simulink model "ClosedLoopControl"  (R2016b)
settings: Solver=FixedStepDiscrete  StartTime=0.0  StopTime=Inf  FixedStep=sCoreParams.core.stepPeriod  RelTol=1e-3  EnableMultiTasking=on
undefined symbols (not defined in the file): fdesignblkfcn, gcbh, High, sCoreParams, sCoreParams_decoders_chanceDetector_randStimEventsPerSec, sCoreParams_decoders_txDetector_channel1, sCoreParams_decoders_txDetector_channel2, sCoreParams_decoders_txDetector_detectChannelInds, sCoreParams_decoders_txDetector_nChannels, sCoreParams_Features_Baseline_initialThresholdValue, sCoreParams_Features_Baseline_weightPreviousThreshold, sCoreParams_Features_Data_SmoothWindowsDurationSamples, sCoreParams_stimulator_stimAfterDelaySteps
libraries: dsparch4 x20, dspstat3 x19, dspspect3 x6, dspfdesign x2, dspindex x2, dspswit3 x1
(part 4 of 6)

== system ClosedLoopControl/FilterBanks/Variant FILTER 1000/8-15Hz Alpha FIR ==
  EEGData : Inport
  Generated Filter Block : DiscreteFir  Tag=BlockMethodSubSystem  Coefficients=[1.1166843982614926e-06 -5.1505963497875887e-06 -1.2812602333555129e-05 -2.1871054990882468e-05 -3.2323373818540652e-05 -4.4162634838047868e-05 -5.7377540676991869e-05 -7.195240245586386e-05 -8.7867133639842035e-05 -0.00010509725598372113 -0.00012361391766630315 -0.00014338392367813367 -0.000164369778493665 -0.00018652974102566303 -0.00020981789182618625 -0.0002341842124648283 -0.0002595746769810637 -0.00028593135527383055 -0.00031319252825774447 -0.00034129281458180586 -0.00037016330867327857 -0.00039973172983648352 -0.00042992258210380332 -0.00046065732450443646 -0.00049185455138502153 -0.00052343018238589314 -0.000555297661646971 -0.0005873681657885076 -0.00061955082018408858 -0.00065175292301663287 -0.00068388017658249981 -0.00071583692528446631 -0.00074752639973140443 -0.00077885096634068161 -0.00080971238181931681 -0.00084001205188102607 -0.00086965129353934944 -0.00089853160030159028 -0.0009265549095744043 -0.00095362387157998788 -0.00097964211907159478 -0.0010045145371285577 -0.0010281475323047058 -0.0010504493003992363 -0.0010713300921165658 -0.0010907024758808866 -0.0011084815970723843 -0.0011245854329553625 -0.00113893504257369 -0.0011514548108961891 -0.001162072686503848 -0.0011707204121218695 -0.0011773337473127315 -0.0011818526826615754 -0.0011842216448022078 -0.0011843896916509528 -0.0011823106972363748 -0.0011779435255354414 -0.00117125219275111 -0.0011622060174923557 -0.0011507797583454361 -0.001136953738354511 -0.0011207139559606311 -0.0011020521819804436 -0.0010809660422397137 -0.001057459085511797 -0.0010315408364474827 -0.0010032268332200427 -0.00097253864964778316 -0.00093950390159584351 -0.00090415623749921738 -0.00086653531289007147 -0.00082668674885407638 -0.00078466207438273922 -0.00074051865263137029 -0.00069431959113537079 -0.0006461336360806941 -0.00059603505076769926 -0.00054410347845094465 -0.00049042378978056769 -0.0004350859151140158 -0.00037818466200922462 -0.0003198195182527428 -0.00026009444081761201 -0.00019911763118664756 -0.00013700129751690498 -7.3861404160011573e-05 -9.8174090911267554e-06 5.5008010163797022e-05 0.00012048924147724876 0.00018649803328639865 0.00025290379928409514 0.00031957393191114501 0.00038637412389685354 0.00045316869706702476 0.00051982093761261162 0.00058619343698820684 0.00065214843758748075 0.00071754818232275524 0.00078225526721801533 0.00084613299610908864 0.00090904573653135254 0.00097085927586427958 0.0010314411767934721 0.0010906611311446244 0.0011483913111399052 0.0012045067171260633 0.0012588855208245753 0.0013114094031579228 0.0013619638857121615 0.0014104386549047448 0.0014567278779377545 0.0015007305096304167 0.0015423505892410412 0.0015814975264072709 0.001618086375354588 0.0016520380965466808 0.0016832798049771526 0.0017117450043303123 0.0017373738062692796 0.0017601131341423238 0.0017799169104332252 0.0017967462273182613 0.0018105694997313348 0.0018213626003794627 0.0018291089761933916 0.0018337997457423454 0.0018354337771877447 0.0018340177463980255 0.0018295661748954481 0.0018221014473556757 0.0018116538084320456 0.0017982613387285684 0.0017819699097986867 0.0017628331181006056 0.0017409121978943678 0.0017162759131207782 0.0016890004283574528 0.0016591691590027344 0.0016268726008937253 0.001592208139620101 0.0015552798398505627 0.0015161982150436648 0.0014750799779690521 0.0014320477725188181 0.0013872298873415828 0.0013407599518838245 0.0012927766154738488 0.001243423210133381 0.0011928473978500983 0.0011412008030911467 0.0010886386313827949 0.0010353192748249133 0.00098140390545031655 0.0009270560573785804 0.00087244119875139019 0.00081772629447154682 0.00076307936080061199 0.00070866901290059193 0.00065466400643282975 0.00060123277435255879 0.00054854296006001896 0.00049676094808876381 0.00044605139352870261 0.00039657675139517979 0.00034849680716653192 0.0003019682097202846 0.00025714400790310016 0.00021417319197122785 0.00017320024113676101 0.00013436467845048239 9.7800634244212941e-05 6.3636419344704006e-05 3.1994109256920648e-05 ...(+13836 chars)]  InputProcessing=Columns as channels (frame based)
  filteredData : Outport
  wires:
  EEGData/1 -> Generated Filter Block/1
  Generated Filter Block/1 -> filteredData/1

== system ClosedLoopControl/FilterBanks/Variant FILTER 1000/8-15Hz Alpha IIR ==
  EEGData : Inport
  Generated Filter Block : dsparch4/Biquad Filter  Tag=BlockMethodSubSystem  IIRFiltStruct=Direct form II  CoeffSource=Specify via dialog  BiQuadCoeffs=[0.03152382825305871 0 -0.03152382825305871 1 -1.9684345944585124 0.97712907102407076;0.025560463242853482 0 -0.025560463242853482 1 -1.9681378422909206 0.97119496912467995;0.024051049006500725 0 -0.024051049006500725 1 -1.9527425358453594 0.95696285762488253;0.007268915115754877 0 -0.007268915115754877 1 -1.9493011946808791 0.95637402951036332;0.026129757567963516 0 -0.026129757567963516 1 -1.9934192573086764 0.99586503566620033;0.017980975322089195 0 -0.017980975322089195 1 -1.9829215784521332 0.99203325429180822;0.032745837103951347 0 -0.032745837103951347 1 -1.9568602017984618 0.9648466951679141;0.029923094077486778 0 -0.029923094077486778 1 -1.9599295286379477 0.96347484474396472;0.027004967888092691 0 -0.027004967888092691 1 -1.9477670142381809 0.95284532685210388;0.032600500740339038 0 -0.032600500740339038 1 -1.9463207424125604 0.9523841483440838;0.01817150925319717 0 -0.01817150925319717 1 -1.9850778884335281 0.98761149045414087;2 0 -2 1 -1.9766276718191218 0.97935766676512392]  a0Flag=Warning  IC=0  ICnum=0  ICden=0  InputProcessing=Columns as channels (frame based)  denAccumFracLength=30  denProdOutputFracLength=30  secondMemoryFracLength=15  roundingMode=Floor  overflowMode=off  ScaleValues=[0.0021262776362185819;1;1;1;1;1;1;1;1;1;1;1;4.7772804403775435]  optimizeScaleValues=off  ScaleValueMode=Specify via input port (g)  scaleValueFracLength=14  FilterSource=Specify via dialog  FilterObject=BQF
  filteredData : Outport
  wires:
  EEGData/1 -> Generated Filter Block/1
  Generated Filter Block/1 -> filteredData/1

== system ClosedLoopControl/FilterBanks/Variant FILTER 1000/80-200Hz HFORipple FIR ==
  EEGData : Inport
  Generated Filter Block : DiscreteFir  Tag=BlockMethodSubSystem  Coefficients=[-0.029929468383316192 0.027584903344857116 0.006558984880081789 -0.0071603267655065833 -0.013247180355273648 -0.013135920645701411 -0.0090343519140387157 -0.0032754151064268641 0.0022272516299482945 0.0061526392461596219 0.0079390912269469774 0.0076686887032404866 0.0060227556600073798 0.0039349955485136062 0.002396304305429954 0.0020527359637715833 0.0031029488412524647 0.0051247167458305515 0.0073477544104056103 0.0087957682525686351 0.0088043284423398316 0.00710059570242208 0.0041318613604908808 0.00067350576530127854 -0.0021332528816080248 -0.0036147405910317496 -0.0034016416976209995 -0.001904243925895048 -9.8116221945575288e-05 0.0011838227951950983 0.0010052402801807789 -0.00069375398602379568 -0.0033161108088197999 -0.0058093921651041838 -0.0070688296122434977 -0.0062279411320784531 -0.0032465358048272691 0.0011033746367409905 0.0054903794295953143 0.0085941785365106216 0.0095047981352248956 0.0081292793472463598 0.005237259579484288 0.0022388728520793405 0.00053886046527349546 0.00096339401712913775 0.0033698853216399469 0.006695473988653354 0.0093294470183197739 0.009730061973901652 0.0070986567584101143 0.0017181031971334401 -0.0049383095140956221 -0.010887765954854724 -0.014221289453944019 -0.013976819805220315 -0.010530893082807774 -0.0054287582554014349 -0.00088011910410184385 0.0011679539587099719 -0.00014547643883787431 -0.0041760754011632081 -0.008944366661674398 -0.011801424674010449 -0.010562162379392094 -0.0044555321547889229 0.0053958544645990661 0.016263138140394436 0.024694650965907963 0.027841496662202841 0.024596298085779726 0.016203929024829047 0.0058734470287940752 -0.0023244041555813555 -0.0050790680728182019 -0.0012630785826390906 0.0072633206754821183 0.016070445540513408 0.019596048919655211 0.013222985157710941 -0.0046438574372398012 -0.031492102130720984 -0.060763349522214613 -0.083541115124259574 -0.09120184118086383 -0.078307752643135484 -0.04470543854444764 0.0038254224665319886 0.056784017626830177 0.10164096275331343 0.12730747905853101 0.12730747905853101 0.10164096275331343 0.056784017626830177 0.0038254224665319886 -0.04470543854444764 -0.078307752643135484 -0.09120184118086383 -0.083541115124259574 -0.060763349522214613 -0.031492102130720984 -0.0046438574372398012 0.013222985157710941 0.019596048919655211 0.016070445540513408 0.0072633206754821183 -0.0012630785826390906 -0.0050790680728182019 -0.0023244041555813555 0.0058734470287940752 0.016203929024829047 0.024596298085779726 0.027841496662202841 0.024694650965907963 0.016263138140394436 0.0053958544645990661 -0.0044555321547889229 -0.010562162379392094 -0.011801424674010449 -0.008944366661674398 -0.0041760754011632081 -0.00014547643883787431 0.0011679539587099719 -0.00088011910410184385 -0.0054287582554014349 -0.010530893082807774 -0.013976819805220315 -0.014221289453944019 -0.010887765954854724 -0.0049383095140956221 0.0017181031971334401 0.0070986567584101143 0.009730061973901652 0.0093294470183197739 0.006695473988653354 0.0033698853216399469 0.00096339401712913775 0.00053886046527349546 0.0022388728520793405 0.005237259579484288 0.0081292793472463598 0.0095047981352248956 0.0085941785365106216 0.0054903794295953143 0.0011033746367409905 -0.0032465358048272691 -0.0062279411320784531 -0.0070688296122434977 -0.0058093921651041838 -0.0033161108088197999 -0.00069375398602379568 0.0010052402801807789 0.0011838227951950983 -9.8116221945575288e-05 -0.001904243925895048 -0.0034016416976209995 -0.0036147405910317496 -0.0021332528816080248 0.00067350576530127854 0.0041318613604908808 0.00710059570242208 0.0088043284423398316 0.0087957682525686351 0.0073477544104056103 0.0051247167458305515 0.0031029488412524647 0.0020527359637715833 0.002396304305429954 0.0039349955485136062 0.0060227556600073798 0.0076686887032404866 0.0079390912269469774 0.0061526392461596219 0.0022272516299482945 -0.0032754151064268641 -0.0090343519140387157 -0.013135920645701411 -0.013247180355273648 -0.0071603267655065833 0.006558984880081789 0.027584903344857116 -0.029929468383316192]  InputProcessing=Columns as channels (frame based)
  filteredData : Outport
  wires:
  EEGData/1 -> Generated Filter Block/1
  Generated Filter Block/1 -> filteredData/1

== system ClosedLoopControl/FilterBanks/Variant FILTER 1000/80-200Hz HFORipple IIR ==
  EEGData : Inport
  Generated Filter Block : dsparch4/Biquad Filter  Tag=BlockMethodSubSystem  IIRFiltStruct=Direct form II  CoeffSource=Specify via dialog  BiQuadCoeffs=[0.50528002861034449 0 -0.50528002861034449 1 -0.53665660289882711 0.75825785021660019;0.37399875098270552 0 -0.37399875098270552 1 -1.4711915314319288 0.71332426960135642;0.32821275057331467 0 -0.32821275057331467 1 -1.0345186757915159 0.43765324877783934;0.29499676491259791 0 -0.29499676491259791 1 -0.69551179724291168 0.41191642538380135;0.32493798324944001 0 -0.32493798324944001 1 -1.2744782347700396 0.5651630856467672;0.12068212430570054 0 -0.12068212430570054 1 -0.57105344445275907 0.53488062009913828;0.30353084173161105 0 -0.30353084173161105 1 -1.7216581336938179 0.9551476738605682;0.49261556542327029 0 -0.49261556542327029 1 -0.55816431380313891 0.91150109211215435;0.18405150815598884 0 -0.18405150815598884 1 -1.3775879521174472 0.63826277797818964;0.38868856803283353 0 -0.38868856803283353 1 -0.54207706836534775 0.63362507430418646;0.35661452914905484 0 -0.35661452914905484 1 -0.90735390108977221 0.39967170660663376;0.43873431466398466 0 -0.43873431466398466 1 -0.79136443478105378 0.39064255793275482;0.28072258344311274 0 -0.28072258344311274 1 -1.1597022390795022 0.49621962903073175;0.54469763526328785 0 -0.54469763526328785 1 -0.62218168437391907 0.46078823772386801;0.27221303222116677 0 -0.27221303222116677 1 -1.6408415799416185 0.87038248002913765;0.99524691708840851 0 -0.99524691708840851 1 -1.5580903198942666 0.79034416212980196]  a0Flag=Warning  IC=0  ICnum=0  ICden=0  InputProcessing=Columns as channels (frame based)  denAccumFracLength=30  denProdOutputFracLength=30  secondMemoryFracLength=15  roundingMode=Floor  overflowMode=off  ScaleValues=[0.22997867729739599;1;1;1;1;1;1;1;1;1;1;1;1;1;1;1;1]  optimizeScaleValues=off  ScaleValueMode=Specify via input port (g)  scaleValueFracLength=14  FilterSource=Specify via dialog  FilterObject=BQF
  filteredData : Outport
  wires:
  EEGData/1 -> Generated Filter Block/1
  Generated Filter Block/1 -> filteredData/1

== system ClosedLoopControl/FilterBanks/Variant FILTER 1000/AllBand ==
  EEGData : Inport
  filteredData : Outport
  wires:
  EEGData/1 -> filteredData/1

== system ClosedLoopControl/FilterBanks/Variant FILTER 1000/VariableFreq FIR ==
  EEGData : Inport
  Discrete FIR Filter : DiscreteFir  FilterStructure=Direct form symmetric  Coefficients=sCoreParams.filter.Hd.Numerator
  filteredData : Outport
  wires:
  Discrete FIR Filter/1 -> filteredData/1
  EEGData/1 -> Discrete FIR Filter/1

== system ClosedLoopControl/FilterBanks/Variant FILTER 2000/11-15HZ Spindles IIR ==
  EEGData : Inport
  Generated Filter Block : dsparch4/Biquad Filter  Tag=BlockMethodSubSystem  IIRFiltStruct=Direct form II  CoeffSource=Specify via dialog  BiQuadCoeffs=[2 0 -2 1 -1.9860801464214457 0.987727843501902569]  a0Flag=Warning  IC=0  ICnum=0  ICden=0  InputProcessing=Columns as channels (frame based)  denAccumFracLength=30  denProdOutputFracLength=30  secondMemoryFracLength=15  roundingMode=Floor  overflowMode=off  ScaleValues=[0.000493888847219880567;6.21200325092265171]  optimizeScaleValues=off  ScaleValueMode=Specify via input port (g)  scaleValueFracLength=14  FilterSource=Specify via dialog  FilterObject=BQF
  filteredData : Outport
  wires:
  EEGData/1 -> Generated Filter Block/1
  Generated Filter Block/1 -> filteredData/1

== system ClosedLoopControl/FilterBanks/Variant FILTER 2000/140-200Hz Ripple IIR ==
  EEGData : Inport
  Generated Filter Block : dsparch4/Biquad Filter  Tag=BlockMethodSubSystem  IIRFiltStruct=Direct form II  CoeffSource=Specify via dialog  BiQuadCoeffs=[0.12352657209800035 0 -0.12352657209800035 1 -1.6311590352784913 0.84123752914815553;0.027358370011554025 0 -0.027358370011554025 1 -1.5252134710057248 0.81657832066238856;0.2331538241948424 0 -0.2331538241948424 1 -1.7807649144635369 0.96270781905622915;0.12590142538731877 0 -0.12590142538731877 1 -1.5663146910613774 0.94768937106864404;0.052873711371256564 0 -0.052873711371256564 1 -1.5661160326969752 0.81142026924756905;0.19282809609473742 0 -0.19282809609473742 1 -1.7059346694081983 0.89485388869806892;1.130694590069905 0 -1.130694590069905 1 -1.5227265486047719 0.86313533616119298]  a0Flag=Warning  IC=0  ICnum=0  ICden=0  InputProcessing=Columns as channels (frame based)  denAccumFracLength=30  denProdOutputFracLength=30  secondMemoryFracLength=15  roundingMode=Floor  overflowMode=off  ScaleValues=[0.072632038243158975;1;1;1;1;1;1;1]  optimizeScaleValues=off  ScaleValueMode=Specify via input port (g)  scaleValueFracLength=14  FilterSource=Specify via dialog  FilterObject=BQF
  filteredData : Outport
  wires:
  EEGData/1 -> Generated Filter Block/1
  Generated Filter Block/1 -> filteredData/1

== system ClosedLoopControl/FilterBanks/Variant FILTER 2000/145-200Hz Ripple FIR ==
  EEGData : Inport
  Generated Filter Block : DiscreteFir  Tag=BlockMethodSubSystem  Coefficients=[-0.030781520603345755 0.029736587613204871 0.016279349881715796 0.0078304734697767775 0.0034101124575861563 0.0021109050937578866 0.0029359501791036482 0.0048221357516104943 0.0066675765400677559 0.0075439573200530088 0.0068299029664432159 0.0044170245691875151 0.0007305503624317547 -0.0033144418142821638 -0.0066073626352400397 -0.008115382277290431 -0.007299157247865555 -0.0042500768030829042 0.0001902291282893237 0.0047615272618279983 0.0080537753119725719 0.0090888577269477855 0.007501544338330314 0.0038465594631155176 -0.00074048500280713553 -0.0048863103096512331 -0.0072169181698771429 -0.0073994531081829351 -0.0054270557962657132 -0.002254737434171504 0.00086546613635283404 0.0029149802832981117 0.0034583853146492802 0.0026234557641752754 0.001164732411809373 5.1783863659192464e-05 2.3369551283396184e-05 0.0011599107816354856 0.0028744791094547709 0.004135969419948364 0.0039639887525646025 0.0018331530274210903 -0.0019498921461991101 -0.0062991090714655182 -0.0096028435909793972 -0.010407292076703323 -0.0079421078421768043 -0.0026102640831030394 0.0041590394472750397 0.010237281364097572 0.013611983265214941 0.013116126210911384 0.0087781592628307439 0.0020124063186148997 -0.005021276797438759 -0.010123284187206115 -0.011821380571436675 -0.0099304545038921554 -0.0055932597013606603 -0.00071349819259146352 0.0028002388976299947 0.0038275185978517978 0.0025285946144394666 0.00024688745347431484 -0.0011164507549987698 -3.8298925510396598e-05 0.0038051022729689021 0.00918952477604211 0.013626718379269272 0.014320948674260946 0.009371767654852238 -0.0011215127004242931 -0.014722781888086886 -0.02711168652799726 -0.033490181243977103 -0.030255934127276694 -0.016584097409115692 0.0047929614203095217 0.02810395806549059 0.046075325861400326 0.052266726383597022 0.04336162944653018 0.020556639691233745 -0.010420977616046684 -0.040753154116921785 -0.06119608459496325 -0.065000080365273327 -0.050152269558981596 -0.020277362294476072 0.016311587571896234 0.049020798279318864 0.068226011237433576 0.068226011237433576 0.049020798279318864 0.016311587571896234 -0.020277362294476072 -0.050152269558981596 -0.065000080365273327 -0.06119608459496325 -0.040753154116921785 -0.010420977616046684 0.020556639691233745 0.04336162944653018 0.052266726383597022 0.046075325861400326 0.02810395806549059 0.0047929614203095217 -0.016584097409115692 -0.030255934127276694 -0.033490181243977103 -0.02711168652799726 -0.014722781888086886 -0.0011215127004242931 0.009371767654852238 0.014320948674260946 0.013626718379269272 0.00918952477604211 0.0038051022729689021 -3.8298925510396598e-05 -0.0011164507549987698 0.00024688745347431484 0.0025285946144394666 0.0038275185978517978 0.0028002388976299947 -0.00071349819259146352 -0.0055932597013606603 -0.0099304545038921554 -0.011821380571436675 -0.010123284187206115 -0.005021276797438759 0.0020124063186148997 0.0087781592628307439 0.013116126210911384 0.013611983265214941 0.010237281364097572 0.0041590394472750397 -0.0026102640831030394 -0.0079421078421768043 -0.010407292076703323 -0.0096028435909793972 -0.0062991090714655182 -0.0019498921461991101 0.0018331530274210903 0.0039639887525646025 0.004135969419948364 0.0028744791094547709 0.0011599107816354856 2.3369551283396184e-05 5.1783863659192464e-05 0.001164732411809373 0.0026234557641752754 0.0034583853146492802 0.0029149802832981117 0.00086546613635283404 -0.002254737434171504 -0.0054270557962657132 -0.0073994531081829351 -0.0072169181698771429 -0.0048863103096512331 -0.00074048500280713553 0.0038465594631155176 0.007501544338330314 0.0090888577269477855 0.0080537753119725719 0.0047615272618279983 0.0001902291282893237 -0.0042500768030829042 -0.007299157247865555 -0.008115382277290431 -0.0066073626352400397 -0.0033144418142821638 0.0007305503624317547 0.0044170245691875151 0.0068299029664432159 0.0075439573200530088 0.0066675765400677559 0.0048221357516104943 0.0029359501791036482 0.0021109050937578866 0.0034101124575861563 0.0078304734697767775 0.016279349881715796 0.029736587613204871 -0.030781520603345755]  InputProcessing=Columns as channels (frame based)
  filteredData : Outport
  wires:
  EEGData/1 -> Generated Filter Block/1
  Generated Filter Block/1 -> filteredData/1

== system ClosedLoopControl/FilterBanks/Variant FILTER 2000/15-30Hz Beta FIR ==
  EEGData : Inport
  Generated Filter Block : DiscreteFir  Tag=BlockMethodSubSystem  Coefficients=[0.00024932604967076838 0.00022562835097991477 0.00020055883023604209 0.00017450536010432124 0.00014787470676203059 0.00012108823390752595 9.4577357124501601e-05 6.8778794034300684e-05 4.4129658786645323e-05 2.1062452077078791e-05 -2.7492423039110665e-19 -1.8649603383242571e-05 -3.4497993888248867e-05 -4.7181419195105332e-05 -5.6365448928950234e-05 -6.1749457622014875e-05 -6.3070826807644178e-05 -6.0108814576680591e-05 -5.2688043611973456e-05 -4.0681561988766557e-05 -2.401343486143125e-05 -2.6608295179705497e-06 2.3344438865809144e-05 5.3914928145513692e-05 8.8907178484600832e-05 0.00012812192564416256 0.00017130492763639147 0.00021814840757232323 0.00026829310886882917 0.00032133095223859563 0.0003768082771425536 0.00043422964371071202 0.00049306216460859417 0.00055274033001634403 0.00061267128286881189 0.00067224049584787074 0.00073081779639075947 0.00078776368124497246 0.00084243585792020525 0.00089419594681682153 0.00094241627489654754 0.00098648668954764637 0.0010258213198195128 0.0010598652114882623 0.0010881007624864356 0.0011100538860983283 0.0011252998309913629 0.0011334685896186197 0.0011342498297744687 0.0011273972880916526 0.0011127325690035576 0.0010901482981200605 0.0010596105850321073 0.0010211607572136851 0.0009749163338677976 0.00092107121619643812 0.00085989507858800552 0.0007917319535292195 0.00071699801157699126 0.000636178546380586 0.00054982418343449066 0.00045854633987444526 0.00036301197110909526 0.00026393764831425211 0.00016208301871255902 5.8243708028869324e-05 -4.6756268537101536e-05 -0.00015207251412670736 -0.00025684859845693733 -0.00036022466317640564 -0.00046134619693138701 -0.00055937288948681779 -0.00065348747192239289 -0.00074290444855744885 -0.00082687862588018109 -0.00090471334438626367 -0.00097576832087874178 -0.0010394670114429023 -0.0010953034089747223 -0.0011428481937856628 -0.0011817541613957556 -0.0012117608581163283 -0.0012326983623577709 -0.001244490157711635 -0.0012471550526754304 -0.0012408081113295473 -0.0012256605692480087 -0.0012020187193297893 -0.0011702817629714256 -0.0011309386329549156 -0.0010845638054844833 -0.001031812129855466 -0.0009734127151604698 -0.00091016192411399002 -0.00084291553438961802 -0.00077258013769825561 -0.00070010385607981835 -0.00062646646342703839 -0.0005526690080073168 -0.0004797230386016781 -0.00040863954275302474 -0.00034041771043132122 -0.00027603364011376626 -0.00021642910678700521 -0.00016250051266128044 -0.00011508814141064184 -7.4965835499315943e-05 -4.2831213615604891e-05 -1.9296541418413303e-05 -4.8803637284107098e-06 -1.5115631016753627e-19 -4.9649974395269964e-06 -1.9971627550228426e-05 -4.5098502258702979e-05 -8.0303375196634768e-05 -0.00012542118227197094 -0.0001801633634729392 -0.00024411849502299244 -0.00031675424767009996 -0.00039742067318219532 -0.00048535480717015462 -0.00057968656231336378 -0.00067944587206669998 -0.00078357103112883036 -0.00089091816549832607 -0.0010002717519816938 -0.0011103560946900746 -0.0012198476545067958 -0.0013273881168597975 -0.0014315980735153974 -0.0015310911856396493 -0.0016244886881564714 -0.00171043408956193 -0.0017876079169135538 -0.0018547423527700514 -0.0019106356094641382 -0.0019541658862868043 -0.0019843047569679832 -0.0020001298382613876 -0.0020008365954695844 -0.0019857491473510187 -0.0019543299409892647 -0.0019061881768149373 -0.0018410868749752605 -0.001758948486552175 -0.0016598589666296502 -0.0015440702407827466 -0.0014120010120704913 -0.0012642358719159457 -0.0011015226951933369 -0.00092476831724877333 -0.00073503250828539982 -0.00053352027836815253 -0.0003215725640653392 -0.00010065536526088647 0.00012765258224192586 0.00036167349622888341 0.00059964548191373797 0.00083973857760329443 0.0010800717660899655 0.0013187307933636354 0.0015537866253548353 0.0017833143641044383 0.0020054124371196732 0.0022182218678259581 0.0024199454310448224 0.0026088664953892731 0.0027833673544188494 0.002941946850368166 0.0030832370982642947 0.0032060191242710254 0.0033092372401093842 0.00339201198535369 ...(+10128 chars)]  InputProcessing=Columns as channels (frame based)
  filteredData : Outport
  wires:
  EEGData/1 -> Generated Filter Block/1
  Generated Filter Block/1 -> filteredData/1
